simulink model "PenduloDoble_PD_clasico"  (R2013a)
settings: Solver=ode3  StartTime=0.0  StopTime=300  FixedStep=0.01  RelTol=1e-3
undefined symbols (not defined in the file): g, Theta1, Theta2, Theta3, Theta4, Theta5
libraries: mblibv1 x12
settings Model: Creator=LornBaltymor  LastModifiedBy=Daniel
settings SimMechanicsCC: VisOnUpdateDiagram=on  VisDuringSimulation=on

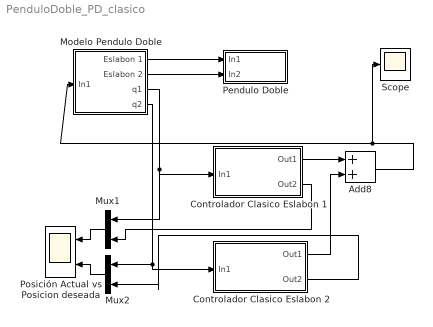
== system PenduloDoble_PD_clasico ==
  Add8 : Sum
  Controlador Clasico Eslabon 1 : Subsystem
  Controlador Clasico Eslabon 2 : Subsystem
  Modelo Pendulo Doble : Subsystem
  Mux1 : Mux  Inputs=2
  Mux2 : Mux  Inputs=2
  Pendulo Doble : Subsystem
  Posición Actual vs Posicion deseada : Scope  NumInputPorts=2
      settings: TimeRange=15  YMin=-2.5~0  YMax=3.25~6  SaveName=ScopeData4
  Scope : Scope
      settings: SaveName=Control
  wires:
  Add8/1 -> Scope/1, Modelo Pendulo Doble/1(In1)
  Modelo Pendulo Doble/1(Eslabon 1) -> Pendulo Doble/1(In1)
  Modelo Pendulo Doble/2(Eslabon 2) -> Pendulo Doble/2(In2)
  Modelo Pendulo Doble/3(q1) -> Mux1/1, Controlador Clasico Eslabon 1/1(In1)
  Modelo Pendulo Doble/4(q2) -> Mux2/1, Controlador Clasico Eslabon 2/1(In1)
  Mux2/1 -> Posición Actual vs Posicion deseada/2
  Mux1/1 -> Posición Actual vs Posicion deseada/1
  Controlador Clasico Eslabon 2/1(Out1) -> Add8/2
  Controlador Clasico Eslabon 2/2(Out2) -> Mux2/2
  Controlador Clasico Eslabon 1/1(Out1) -> Add8/1
  Controlador Clasico Eslabon 1/2(Out2) -> Mux1/2

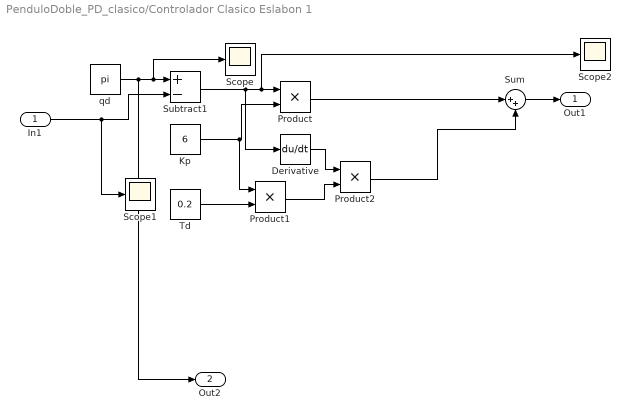
== system PenduloDoble_PD_clasico/Controlador Clasico Eslabon 1 ==
  In1 : Inport
  Derivative : Derivative
  Kp : Constant  Value=6
  Product : Product
  Product1 : Product
  Product2 : Product
  Scope : Scope
      settings: SaveName=Referencia
  Scope1 : Scope
      settings: SaveName=Posi
  Scope2 : Scope
      settings: SaveName=Error1
  Subtract1 : Sum  Inputs=+-
  Sum : Sum  Inputs=|++
  Td : Constant  Value=0.2
  qd : Constant  Value=pi
  Out1 : Outport
  Out2 : Outport  Port=2
  wires:
  In1/1 -> Scope1/1, Subtract1/2
  Subtract1/1 -> Derivative/1, Scope2/1, Product/1
  qd/1 -> Out2/1, Scope/1, Subtract1/1
  Kp/1 -> Product1/1, Product/2
  Product/1 -> Sum/1
  Product2/1 -> Sum/2
  Product1/1 -> Product2/2
  Td/1 -> Product1/2
  Derivative/1 -> Product2/1
  Sum/1 -> Out1/1

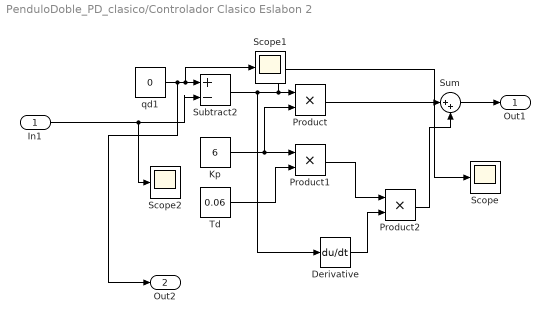
== system PenduloDoble_PD_clasico/Controlador Clasico Eslabon 2 ==
  In1 : Inport
  Derivative : Derivative
  Kp : Constant  Value=6
  Product : Product
  Product1 : Product
  Product2 : Product
  Scope : Scope
      settings: SaveName=Error2
  Scope1 : Scope
      settings: SaveName=Ref1
  Scope2 : Scope
      settings: SaveName=Posi1
  Subtract2 : Sum  Inputs=+-
  Sum : Sum  Inputs=|++
  Td : Constant  Value=0.06
  qd1 : Constant  Value=0
  Out1 : Outport
  Out2 : Outport  Port=2
  wires:
  In1/1 -> Scope2/1, Subtract2/2
  qd1/1 -> Scope1/1, Subtract2/1, Out2/1
  Subtract2/1 -> Derivative/1, Scope/1, Product/1
  Kp/1 -> Product1/1, Product/2
  Td/1 -> Product1/2
  Product1/1 -> Product2/1
  Derivative/1 -> Product2/2
  Product2/1 -> Sum/2
  Product/1 -> Sum/1
  Sum/1 -> Out1/1

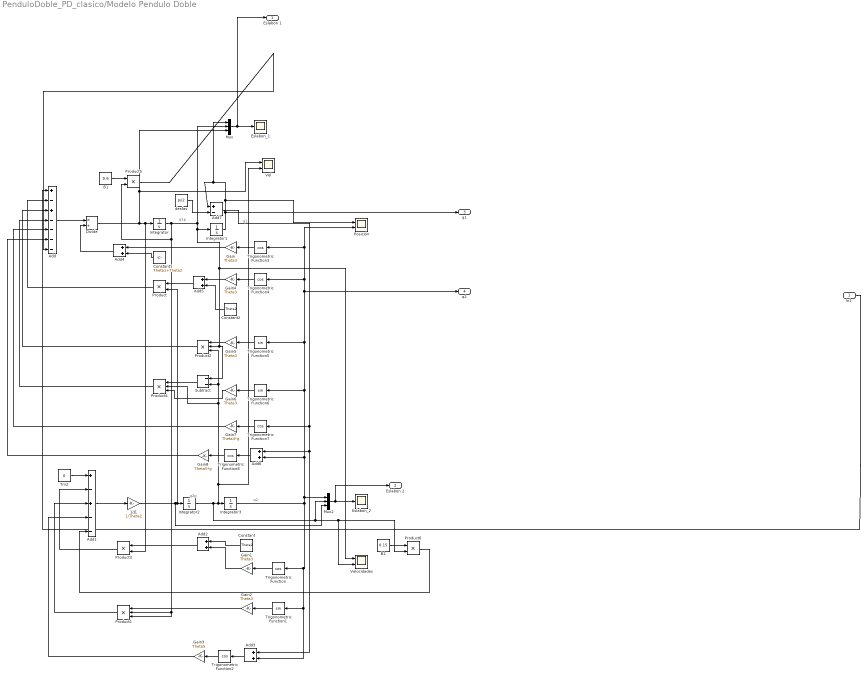
== system PenduloDoble_PD_clasico/Modelo Pendulo Doble ==
  note: q2
  note: q1
  note: q1p
  note: q2p
  In1 : Inport
  1/J1 : Gain  Gain=1/Theta2
  Add : Sum  Inputs=+-+----
  Add1 : Sum  Inputs=+-+--
  Add{2..6} (5 alike) : Sum
  Add7 : Sum  Inputs=+-
  B1 : Constant  Value=0.6
  B2 : Constant  Value=0.15
  Constant : Constant  Value=Theta2
  Constant1 : Constant  Value=Theta1+Theta2
  Constant2 : Constant  Value=Theta2
  Divide : Product  Inputs=*/
  Eslabon_1 : Scope
      settings: YMin=-1000  YMax=12000
  "Eslabon_2 " : Scope
      settings: YMin=-1000  YMax=12000  SaveName=ScopeData2
  Gain{,1..2,4..6} (6 alike) : Gain  Gain=Theta3
  Gain3 : Gain  Gain=Theta5
  Gain7 : Gain  Gain=Theta4*g
  Gain8 : Gain  Gain=Theta5*g
  Integrator{,1..3} (4 alike) : Integrator
  Mux : Mux  Inputs=3
  Mux2 : Mux  Inputs=3
  Posición : Scope  NumInputPorts=2
      settings: YMin=3~-4  YMax=6.5~0.25
  Product{,3,5..6} (4 alike) : Product
  Product1 : Product  Inputs=3
  Product2 : Product  Inputs=3
  Product4 : Product  Inputs=3
  Subtract : Sum  Inputs=--
  Tm2 : Constant  Value=0
  Trigonometric Function{,2..4,7..8} (6 alike) : Trigonometry  Operator=cos
  Trigonometric Function1 : Trigonometry
  Trigonometric Function5 : Trigonometry
  Trigonometric Function6 : Trigonometry
  Vel : Scope  NumInputPorts=2
      settings: YMin=-70~-1.5  YMax=70~1.5  SaveName=ScopeData5
  Velocidades : Scope  NumInputPorts=2
      settings: YMin=-1000~-5  YMax=12000~5  SaveName=ScopeData3
  desfas : Constant  Value=pi/2
  Eslabon 1 : Outport
  Eslabon 2 : Outport  Port=2
  q1 : Outport  Port=3
  q2 : Outport  Port=4
  wires:
  Add1/1 -> 1/J1/1
  1/J1/1 -> Mux2/3, Product/2, Integrator2/1
  Integrator2/1 -> Velocidades/2, Product6/2, Mux2/2, Vel/2, Product4/2, Subtract/2, Product2/3, Integrator3/1
  Divide/1 -> Mux/3, Vel/1, Product3/2, Integrator/1
  Trigonometric Function5/1 -> Gain5/1
  Trigonometric Function4/1 -> Gain4/1
  Product2/1 -> Add/3
  Trigonometric Function/1 -> Gain1/1
  Subtract/1 -> Product4/1
  Gain6/1 -> Product4/3
  Trigonometric Function6/1 -> Gain6/1
  Product4/1 -> Add/4
  Gain5/1 -> Product2/1
  Gain7/1 -> Add/5
  Trigonometric Function7/1 -> Gain7/1
  Constant1/1 -> Add4/2
  Product1/1 -> Add1/3
  Add2/1 -> Product3/1
  Gain3/1 -> Add1/4
  Add3/1 -> Trigonometric Function2/1
  Trigonometric Function3/1 -> Gain/1
  Add/1 -> Divide/1
  Gain2/1 -> Product1/1
  Integrator3/1 -> Mux2/1, q2/1, Trigonometric Function4/1, Trigonometric Function3/1, Posición/2, Trigonometric Function5/1, Trigonometric Function6/1, Add6/2, Add3/2, Trigonometric Function1/1, Trigonometric Function/1
  Gain4/1 -> Add5/1
  Add5/1 -> Product/1
  Trigonometric Function2/1 -> Gain3/1
  Trigonometric Function1/1 -> Gain2/1
  Constant2/1 -> Add5/2
  Product/1 -> Add/2
  Product3/1 -> Add1/2
  Constant/1 -> Add2/1
  Gain1/1 -> Add2/2
  Gain/1 -> Add4/1
  Add4/1 -> Divide/2
  Product5/1 -> Add/7
  Trigonometric Function8/1 -> Gain8/1
  Gain8/1 -> Add/6
  Mux/1 -> Eslabon 1/1, Eslabon_1/1
  desfas/1 -> Add7/2
  B1/1 -> Product5/1
  B2/1 -> Product6/1
  Mux2/1 -> Eslabon 2/1, "Eslabon_2 "/1
  Add6/1 -> Trigonometric Function8/1
  Product6/1 -> Add1/5
  Integrator1/1 -> q1/1, Posición/1, Mux/1, Add7/1
  Tm2/1 -> Add1/1
  Add7/1 -> Trigonometric Function7/1, Add6/1, Add3/1
  In1/1 -> Add/1
  Integrator/1 -> Integrator1/1, Velocidades/1, Subtract/1, Product2/2, Mux/2, Product5/2, Product1/3, Product1/2

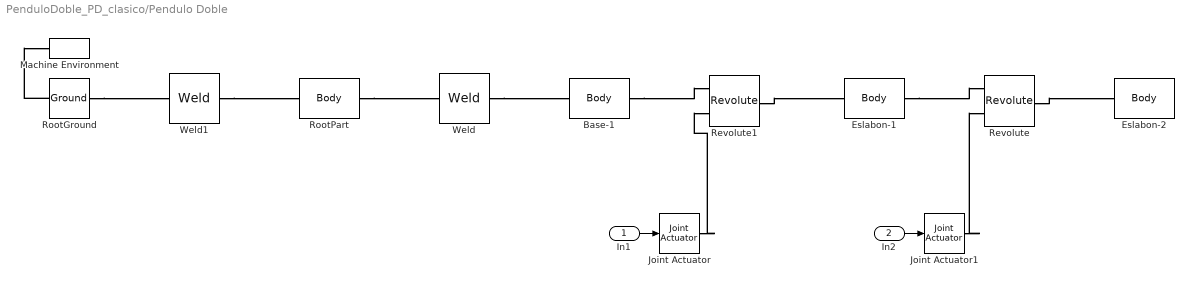
== system PenduloDoble_PD_clasico/Pendulo Doble ==
  In1 : Inport
  In2 : Inport  Port=2
  Base-1 : mblibv1/Bodies/Body  LConnTagsString=CS2  RConnTagsString=CS3  UpdateFromCAD=on  DialogClass=MechanicalBodyBlock  Mass=0.0531084  MassUnits=kg  InertiaUnits=kg*m^2  Inertia=[2.67312e-05,0,0;0,2.67312e-05,0;0,0,5.25773e-05]  Shape=Cylinder  ShapeDims=[1 1]  ShapeUnits=m  ShapeUse=false  Density=1  DensityUnits=kg/m^3  DensityUse=false  GraphicsMode=GFXFILE  GraphicsFileName=PenduloDoble - Base-1.STL  BodyColorSelMode=COLORPALETTE  BodyColor=[0.792157;0.819608;0.933333]  AttachedToCS=CS1  CG=Right$CG$[0.000677469 0.0029357 0.106066]$WORLD$WORLD$m$[1 0 0;0 1 0;0 0 1]$3x3 Transform$rad$WORLD$false$none  WorkingFrames=Right$CS1$[0.000677469 0.0029357 0.101066]$WORLD$WORLD$m$[1 0 0;0 1 0;0 0 1]$3x3 Transform$rad$WORLD$false$none#Left$CS2$[0.000677469 0.0029357 0.106066]$WORLD$WORLD$m$[1 0 0;0 1 0;0 0 1]$3x3 Transform$rad$WORLD$true$none#Right$CS3$[0.000677469 0.0029357 0.111066]$WORLD$WORLD$m$[1 0 0;0 1 0;0 0 1]$3x3 Transform$rad$WORLD$true$none  CGPos=[0.000677469 0.0029357 0.106066]  CGRot=[1 0 0;0 1 0;0 0 1]  CS0Pos=[]  CS0Rot=[]  CS1Pos=[0.000677469 0.0029357 0.101066]  CS1Rot=[1 0 0;0 1 0;0 0 1]  CS2Pos=[0.000677469 0.0029357 0.106066]  CS2Rot=[1 0 0;0 1 0;0 0 1]  CS3Pos=[0.000677469 0.0029357 0.111066]  CS3Rot=[1 0 0;0 1 0;0 0 1]  CS4Pos=[]  CS4Rot=[]  CS5Pos=[]  CS5Rot=[]  CS6Pos=[]  CS6Rot=[]  CS7Pos=[]  CS7Rot=[]  CS8Pos=[]  CS8Rot=[]  CS9Pos=[]  CS9Rot=[]  CS10Pos=[]  CS10Rot=[]  CS11Pos=[]  CS11Rot=[]  CS12Pos=[]  CS12Rot=[]  CS13Pos=[]  CS13Rot=[]  CS14Pos=[]  CS14Rot=[]  CS15Pos=[]  CS15Rot=[]  CS16Pos=[]  CS16Rot=[]  CS17Pos=[]  CS17Rot=[]  CS18Pos=[]  CS18Rot=[]  CS19Pos=[]  CS19Rot=[]  CS20Pos=[]  CS20Rot=[]
  Eslabon-1 : mblibv1/Bodies/Body  LConnTagsString=CS3  RConnTagsString=CS2  UpdateFromCAD=on  DialogClass=MechanicalBodyBlock  Mass=0.0996211  MassUnits=kg  InertiaUnits=kg*m^2  Inertia=[0.000429272,0,0;0,1.78735e-05,0;0,0,0.000445485]  Shape=Cylinder  ShapeDims=[1 1]  ShapeUnits=m  ShapeUse=false  Density=1  DensityUnits=kg/m^3  DensityUse=false  GraphicsMode=GFXFILE  GraphicsFileName=PenduloDoble - Eslabon-1.STL  BodyColorSelMode=COLORPALETTE  BodyColor=[0.792157;0.819608;0.933333]  AttachedToCS=CS1  CG=Right$CG$[0.000565393 -0.0970642 0.116066]$WORLD$WORLD$m$[-0.999999 -0.00112076 0;0.00112076 -0.999999 0;0 0 1]$3x3 Transform$rad$WORLD$false$none  WorkingFrames=Right$CS1$[0.000453317 -0.197064 0.111066]$WORLD$WORLD$m$[-0.999999 -0.00112076 0;0.00112076 -0.999999 0;0 0 1]$3x3 Transform$rad$WORLD$false$none#Right$CS2$[0.000453317 -0.197064 0.121066]$WORLD$WORLD$m$[1 0 0;0 1 0;0 0 1]$3x3 Transform$rad$WORLD$true$none#Left$CS3$[0.000677469 0.0029357 0.111066]$WORLD$WORLD$m$[1 0 0;0 1 0;0 0 1]$3x3 Transform$rad$WORLD$true$none  CGPos=[0.000565393 -0.0970642 0.116066]  CGRot=[-0.999999 -0.00112076 0;0.00112076 -0.999999 0;0 0 1]  CS0Pos=[]  CS0Rot=[]  CS1Pos=[0.000453317 -0.197064 0.111066]  CS1Rot=[-0.999999 -0.00112076 0;0.00112076 -0.999999 0;0 0 1]  CS2Pos=[0.000453317 -0.197064 0.121066]  CS2Rot=[1 0 0;0 1 0;0 0 1]  CS3Pos=[0.000677469 0.0029357 0.111066]  CS3Rot=[1 0 0;0 1 0;0 0 1]  CS4Pos=[]  CS4Rot=[]  CS5Pos=[]  CS5Rot=[]  CS6Pos=[]  CS6Rot=[]  CS7Pos=[]  CS7Rot=[]  CS8Pos=[]  CS8Rot=[]  CS9Pos=[]  CS9Rot=[]  CS10Pos=[]  CS10Rot=[]  CS11Pos=[]  CS11Rot=[]  CS12Pos=[]  CS12Rot=[]  CS13Pos=[]  CS13Rot=[]  CS14Pos=[]  CS14Rot=[]  CS15Pos=[]  CS15Rot=[]  CS16Pos=[]  CS16Rot=[]  CS17Pos=[]  CS17Rot=[]  CS18Pos=[]  CS18Rot=[]  CS19Pos=[]  CS19Rot=[]  CS20Pos=[]  CS20Rot=[]
  Eslabon-2 : mblibv1/Bodies/Body  LConnTagsString=CS2  UpdateFromCAD=on  DialogClass=MechanicalBodyBlock  Mass=0.0996211  MassUnits=kg  InertiaUnits=kg*m^2  Inertia=[0.000429272,0,0;0,1.78735e-05,0;0,0,0.000445485]  Shape=Cylinder  ShapeDims=[1 1]  ShapeUnits=m  ShapeUse=false  Density=1  DensityUnits=kg/m^3  DensityUse=false  GraphicsMode=GFXFILE  GraphicsFileName=PenduloDoble - Eslabon-2.STL  BodyColorSelMode=COLORPALETTE  BodyColor=[0.792157;0.819608;0.933333]  AttachedToCS=CS1  CG=Right$CG$[0.000859131 -0.297063 0.126066]$WORLD$WORLD$m$[-0.999992 0.00405813 0;-0.00405813 -0.999992 0;0 0 1]$3x3 Transform$rad$WORLD$false$none  WorkingFrames=Right$CS1$[0.00126494 -0.397063 0.121066]$WORLD$WORLD$m$[-0.999992 0.00405813 0;-0.00405813 -0.999992 0;0 0 1]$3x3 Transform$rad$WORLD$false$none#Left$CS2$[0.000453317 -0.197064 0.121066]$WORLD$WORLD$m$[1 0 0;0 1 0;0 0 1]$3x3 Transform$rad$WORLD$true$none  CGPos=[0.000859131 -0.297063 0.126066]  CGRot=[-0.999992 0.00405813 0;-0.00405813 -0.999992 0;0 0 1]  CS0Pos=[]  CS0Rot=[]  CS1Pos=[0.00126494 -0.397063 0.121066]  CS1Rot=[-0.999992 0.00405813 0;-0.00405813 -0.999992 0;0 0 1]  CS2Pos=[0.000453317 -0.197064 0.121066]  CS2Rot=[1 0 0;0 1 0;0 0 1]  CS3Pos=[]  CS3Rot=[]  CS4Pos=[]  CS4Rot=[]  CS5Pos=[]  CS5Rot=[]  CS6Pos=[]  CS6Rot=[]  CS7Pos=[]  CS7Rot=[]  CS8Pos=[]  CS8Rot=[]  CS9Pos=[]  CS9Rot=[]  CS10Pos=[]  CS10Rot=[]  CS11Pos=[]  CS11Rot=[]  CS12Pos=[]  CS12Rot=[]  CS13Pos=[]  CS13Rot=[]  CS14Pos=[]  CS14Rot=[]  CS15Pos=[]  CS15Rot=[]  CS16Pos=[]  CS16Rot=[]  CS17Pos=[]  CS17Rot=[]  CS18Pos=[]  CS18Rot=[]  CS19Pos=[]  CS19Rot=[]  CS20Pos=[]  CS20Rot=[]
  Joint Actuator : mblibv1/Sensors &  Actuators/Joint Actuator  UpdateFromCAD=off  PhysicalDomain=Mechanical  PortType=blob  ActuationStyle=Motion  AngleUnits=rad  ArcVelocityUnits=rad/s  ArcAccelerationUnits=rad/s^2  CoordPositionUnits=m  VelocityUnits=m/s  AccelerationUnits=m/s^2  ForceUnits=N  TorqueUnits=N*m  ActiveIO=on  Width=3  DialogClass=MechanicalActuatorBlock  Primitive=R1  ReferenceFrame=Absolute (World)
  Joint Actuator1 : mblibv1/Sensors &  Actuators/Joint Actuator  UpdateFromCAD=off  PhysicalDomain=Mechanical  PortType=blob  ActuationStyle=Motion  AngleUnits=rad  ArcVelocityUnits=rad/s  ArcAccelerationUnits=rad/s^2  CoordPositionUnits=m  VelocityUnits=m/s  AccelerationUnits=m/s^2  ForceUnits=N  TorqueUnits=N*m  ActiveIO=on  Width=3  DialogClass=MechanicalActuatorBlock  Primitive=R1  ReferenceFrame=Absolute (World)
  Machine Environment : mblibv1/Bodies/Machine Environment  PortType=env  PhysicalDomain=Mechanical  DialogTemplateClass=MECH.MachineEnvironment  SyncWhenCopied=off  Gravity=[0 -9.81 0]  GravityUnits=m/s^2  GravityAsSignal=off  Dimensionality=Auto-detect  AnalysisType=Forward dynamics  LinearAssemblyTolerance=1e-3  LinearAssemblyToleranceUnits=m  AngularAssemblyTolerance=1e-3  AngularAssemblyToleranceUnits=rad  ConstraintSolverType=Stabilizing  ConstraintRelTolerance=1e-4  ConstraintAbsTolerance=1e-4  UseRobustSingularityHandling=off  RedundancyAnalysisToleranceType=Automatically select tolerance  RedundancyAnalysisTolerance=1e-14  StatePerturbationType=Fixed  PerturbationSize=1e-5  VisualizeMachine=on  BodyVisualizationType=Use model default body geometries  BodyColorSelMode=Use model default  DefaultBodyColor=[1 0 0]
  Revolute : mblibv1/Joints/Revolute  LConnTagsString=__newl0|SA1  RConnTagsString=__newr0  UpdateFromCAD=on  NumSAPorts=1  CutJoint=off  MarkAsCut=off  Primitives=prismatic  PrimitiveProps=R1$World$[0,0,1]$revolute  DialogClass=JointBlock  R1Axis=[0,0,1]
  Revolute1 : mblibv1/Joints/Revolute  LConnTagsString=__newl0|SA1  RConnTagsString=__newr0  UpdateFromCAD=on  NumSAPorts=1  CutJoint=off  MarkAsCut=off  Primitives=prismatic  PrimitiveProps=R1$World$[0,0,1]$revolute  DialogClass=JointBlock  R1Axis=[0,0,1]
  RootGround : mblibv1/Bodies/Ground  UpdateFromCAD=on  LeftPortType=env  RightPortType=workingframe  PhysicalDomain=Mechanical  DialogClass=GroundBlock  CoordPosition=[0.00070494,-0.154973,0.117909]  CoordPositionUnits=m  StateVectorMgrId=2  MachineId=[3 0]  ShowEnvPort=on
  RootPart : mblibv1/Bodies/Body  LConnTagsString=CS3  RConnTagsString=CS2  UpdateFromCAD=on  DialogClass=MechanicalBodyBlock  Mass=0  MassUnits=kg  InertiaUnits=kg*m^2  Inertia=[0,0,0;0,0,0;0,0,0]  Shape=Cylinder  ShapeDims=[1 1]  ShapeUnits=m  ShapeUse=false  Density=1  DensityUnits=kg/m^3  DensityUse=false  GraphicsMode=MACHINE_DEFAULT  BodyColorSelMode=MACHINE_DEFAULT  BodyColor=[1;0;0]  AttachedToCS=CS1  CG=Right$CG$[0.00070494 -0.154973 0.117909]$WORLD$WORLD$m$[1 0 0;0 1 0;0 0 1]$3x3 Transform$rad$WORLD$false$none  WorkingFrames=Right$CS1$[0 0 0]$WORLD$WORLD$m$[1 0 0;0 1 0;0 0 1]$3x3 Transform$rad$WORLD$false$none#Right$CS2$[0.000677469 0.0029357 0.106066]$WORLD$WORLD$m$[1 0 0;0 1 0;0 0 1]$3x3 Transform$rad$WORLD$true$none#Left$CS3$[0.00070494 -0.154973 0.117909]$WORLD$WORLD$m$[1 0 0;0 1 0;0 0 1]$3x3 Transform$rad$WORLD$true$none  CGPos=[0.00070494 -0.154973 0.117909]  CGRot=[1 0 0;0 1 0;0 0 1]  CS0Pos=[]  CS0Rot=[]  CS1Pos=[0 0 0]  CS1Rot=[1 0 0;0 1 0;0 0 1]  CS2Pos=[0.000677469 0.0029357 0.106066]  CS2Rot=[1 0 0;0 1 0;0 0 1]  CS3Pos=[0.00070494 -0.154973 0.117909]  CS3Rot=[1 0 0;0 1 0;0 0 1]  CS4Pos=[]  CS4Rot=[]  CS5Pos=[]  CS5Rot=[]  CS6Pos=[]  CS6Rot=[]  CS7Pos=[]  CS7Rot=[]  CS8Pos=[]  CS8Rot=[]  CS9Pos=[]  CS9Rot=[]  CS10Pos=[]  CS10Rot=[]  CS11Pos=[]  CS11Rot=[]  CS12Pos=[]  CS12Rot=[]  CS13Pos=[]  CS13Rot=[]  CS14Pos=[]  CS14Rot=[]  CS15Pos=[]  CS15Rot=[]  CS16Pos=[]  CS16Rot=[]  CS17Pos=[]  CS17Rot=[]  CS18Pos=[]  CS18Rot=[]  CS19Pos=[]  CS19Rot=[]  CS20Pos=[]  CS20Rot=[]
  Weld : mblibv1/Joints/Weld  LConnTagsString=__newl0  RConnTagsString=__newr0  UpdateFromCAD=on  NumSAPorts=0  CutJoint=off  MarkAsCut=off  Primitives=weld  PrimitiveProps=W$WORLD$[0.57735,0.57735,0.57735]$weld  DialogClass=JointBlock  WAxis=[0.57735,0.57735,0.57735]
  Weld1 : mblibv1/Joints/Weld  LConnTagsString=__newl0  RConnTagsString=__newr0  UpdateFromCAD=on  NumSAPorts=0  CutJoint=off  MarkAsCut=off  Primitives=weld  PrimitiveProps=W$WORLD$[0.57735,0.57735,0.57735]$weld  DialogClass=JointBlock  WAxis=[0.57735,0.57735,0.57735]
  wires:
  In1/1 -> Joint Actuator/1
  In2/1 -> Joint Actuator1/1
  connections:
  Base-1/RConn1 -- Revolute1/LConn1
  Weld/RConn1 -- Base-1/LConn1
  Weld1/RConn1 -- RootPart/LConn1
  Revolute/RConn1 -- Eslabon-2/LConn1
  Revolute1/RConn1 -- Eslabon-1/LConn1
  RootGround/RConn1 -- Weld1/LConn1
  Eslabon-1/RConn1 -- Revolute/LConn1
  RootGround/LConn1 -- Machine Environment/RConn1
  Joint Actuator/RConn1 -- Revolute1/LConn2
  RootPart/RConn1 -- Weld/LConn1
  Joint Actuator1/RConn1 -- Revolute/LConn2
